simulink model "lti_system"  (R2015a)
settings: Solver=ode4  StartTime=0.0  StopTime=5  FixedStep=0.01  RelTol=1e-3
libraries: cstblocks x1
settings Model: Creator=shohei  LastModifiedBy=shohei

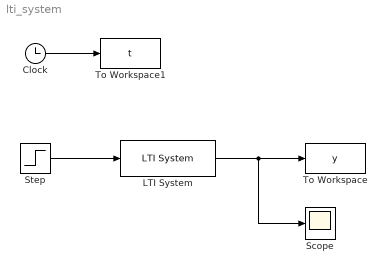
== system lti_system ==
  Clock : Clock
  LTI System : cstblocks/LTI System  sys=sys  IC=x0
  Scope : Scope
  Step : Step  SampleTime=0
  To Workspace : ToWorkspace  VariableName=y  SaveFormat=Timeseries  SampleTime=-1
  To Workspace1 : ToWorkspace  VariableName=t  SaveFormat=Timeseries  SampleTime=-1
  wires:
  Clock/1 -> To Workspace1/1
  Step/1 -> LTI System/1
  LTI System/1 -> Scope/1, To Workspace/1
